simulink model "CBAgent"  (Simulink 7.1)
settings: Solver=ode45  SolverMode=SingleTasking  StartTime=0.0  StopTime=10.0  RelTol=1e-3  AbsTol=1e-6
settings Model: Creator=The MathWorks Inc.  LastModifiedBy=suarezjl  ExtModeTrigMode=oneshot  ExtModeArmWhenConnect=off  ExtModeAutoUpdateStatusClock=off
settings DataIOCC: LimitDataPoints=off  SignalLoggingName=logsOut
settings OptimizationCC: BooleanDataType=off  InlineInvariantSignals=on
settings DebuggingCC: SaveWithParameterizedLinksMsg=none  CheckExecutionContextPreStartOutputMsg=on  CheckExecutionContextRuntimeOutputMsg=on  SignalResolutionControl=TryResolveAllWithWarning  SolverPrmCheckMsg=none  MultiTaskDSMMsg=warning  MultiTaskCondExecSysMsg=none  IntegerOverflowMsg=none  StrictBusMsg=None
settings HardwareCC: TargetUnknown=on
settings ModelReferenceCC: UpdateModelReferenceTargets=IfOutOfDate
settings RTWCC: IncludeERTFirstTime=on
settings GRTTargetCC: TargetFcnLib=ansi_tfl_tmw.mat

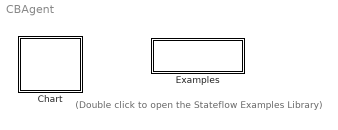
== system CBAgent ==
  note: (Double click to open the
      | Stateflow Examples Library)
  Chart : Stateflow chart
  Examples : Subsystem
      settings: OpenFcn=sf('Private','sf_examples')
      mask Display: disp('Examples')

== system CBAgent/Examples ==

== stateflow chart Chart ==
  state Initialize_Cart
    Aquateen\ControlBasisModule\HP3JCAgent\HP3JC.connect_Initialize()
    Aquateen\ControlBasisModule\HP3JCAgent\HP3JC.servo_ServoOn()
    Aquateen\ControlBasisModule\HP3JCAgent\HP3JC.read_CurrentPosition()
    Aquateen\ControlBasisModule\CartesianCB\CartesianCB.Initialize()
  state MomentForceCB
    Aquateen\ControlBasisModule\HP3JCAgent\HP3JC.read_CurrentPosition()
    Aquateen\ControlBasisModule\MomentForceCB\MomentForceCB.ComputeControlBasis()
    Aquateen\ControlBasisModule\HP3JCAgent\HP3JC.move_JointAngles()
  state \Stop
    Aquateen\ControlBasisModule\HP3JCAgent\HP3JC.connect_Disconnect()
    Aquateen\ControlBasisModule\ForceSensor\StateMachine.Stop()
    Aquateen\ControlBasisModule\ForceSensor\StateMachine.Stop()
  state CartesianCB
    Aquateen\ControlBasisModule\HP3JCAgent\HP3JC.read_CurrentPosition()
    Aquateen\ControlBasisModule\CartesianCB\CartesianCB.ComputeControlBasis()
    Aquateen\ControlBasisModule\HP3JCAgent\HP3JC.move_LinearMotion()
    Aquateen\ControlBasisModule\MomentForceCB\StateMachine.Wait(100)
  state Initialize_MF
    Aquateen\ControlBasisModule\MomentForceCB\MomentForceCB.Initialize()
    Aquateen\ControlBasisModule\ForceSensor\StateMachine.LoadSM()
    Aquateen\ControlBasisModule\ForceSensor\StateMachine.Start()
  (default) -> Initialize_Cart : Start
  Initialize_Cart -> CartesianCB : Always
  MomentForceCB -> MomentForceCB [order 1] : Default
  MomentForceCB -> \Stop [order 2] : Signal="End"
  CartesianCB -> Initialize_MF [order 3] : Signal="Next"
  Initialize_MF -> MomentForceCB : Always
  CartesianCB -> CartesianCB [order 2] : Default
  CartesianCB -> \Stop [order 1] : Signal=End"
